simulink model "ASG_algorithm"  (R2024a)
settings: Solver=ode1  StartTime=0.0  StopTime=60  FixedStep=0.01  RelTol=1e-3
libraries: simulink x3
(part 2 of 3)

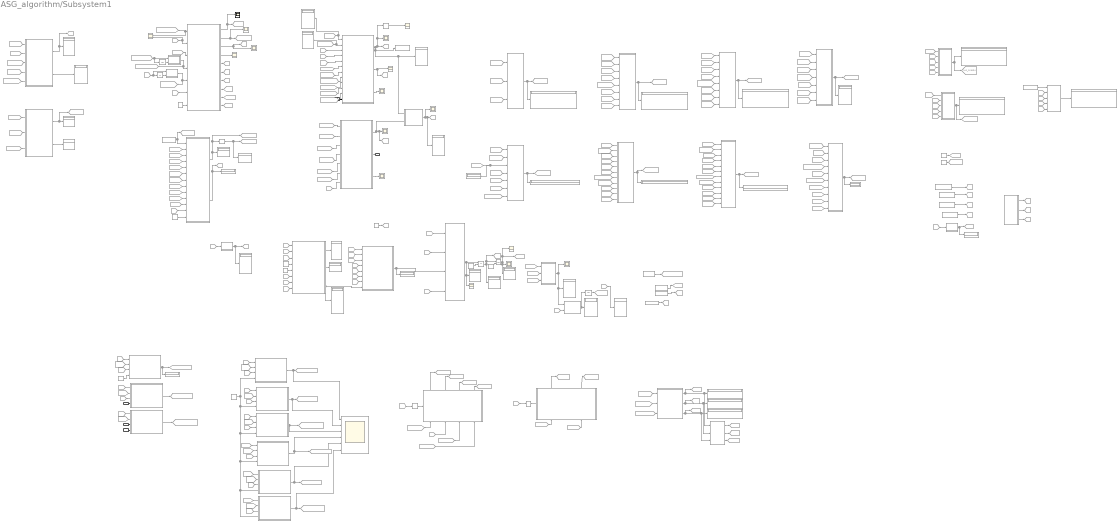
== system ASG_algorithm/Subsystem1 ==
  note: OMEGA DDOT
  note: K matrices
  note: INIT CONDITIONS
      | STEP31
  note: ETA 31
  note: DELTA 3.1
      | DELTA 3.1 DOT
  note: Av. SUBGRADIENT 31
  note: S1
  note: h0(omega_dot)
  note: S31
  note: h0(omega)
  note: CTES motor
  note: h0(x)
  note: ROTATION MATRIX R
  note: R 6x6
  note: THETA3 &
      | ALPHA
  note: DELTA 3.2
      | DELTA 3.2 DOT
  note: G312
  note: G322
  note: G311
  note: G310
  note: G313
  note: G321
  note: G320
  note: G323
  note: S32
  note: ETA 32
  note: INIT CONDITIONS
      | STEP31
  note: S3
  note: Av. SUBGRADIENT 32
  note: OMEGA DDOT
  note: gamma
  note: h3
  note: cte K3
  note: Q constructed
  note: OMEGA DOT
  note: OMEGA
  alpha : Inport
  constant sign : Inport  Port=2
  t : Inport  Port=3
  constant sign1 : Inport  Port=4
  A3 : Scope  Commented=on
  AVERAGE 3 BLOCK : Scope  Commented=on  NumInputPorts=6
  AverageBlock10 : Subsystem  Commented=on
  AverageBlock11 : Subsystem  Commented=on
  AverageBlock12 : Subsystem  Commented=on
  AverageBlock13 : Subsystem  Commented=on
  AverageBlock14 : Subsystem  Commented=on
  AverageBlock6 : Subsystem  Commented=on
  AverageBlock7 : Subsystem  Commented=on
  AverageBlock8 : Subsystem  Commented=on
  AverageBlock9 : Subsystem  Commented=on
  Compare To Constant1 : simulink/Logic and Bit Operations/Compare To Constant  Commented=on  relop===  const=0.0  OutDataTypeStr=boolean
  Compare To Constant2 : simulink/Logic and Bit Operations/Compare To Constant  Commented=on  relop===  const=0.0  OutDataTypeStr=boolean
  Constant11 : Constant  Commented=on  Value=0.5
  Constant12 : Constant  Commented=on  Value=[0;0;0;0;0;0]
  Constant13 : Constant  Commented=on  Value=353
  Constant14 : Constant  Commented=on  Value=2*10^(-4)
  Constant15 : Constant  Commented=on  Value=1.95*10^(-4)  VectorParams1D=off
  Constant17 : Constant  Commented=on  Value=0
  Constant18 : Constant  Commented=on  Value=10
  Constant19 : Constant  Commented=on  Value=[0;0;7;0;0;0]
  Constant{2,6,22,24} (4 alike) : Constant  Commented=on
  Constant20 : Constant  Commented=on  Value=0.00001
  Constant21 : Constant  Commented=on  Value=[0;0;0;0]
  Constant23 : Constant  Commented=on  Value=[1;1;1;1]
  Constant25 : Constant  Commented=on  Value=[0;0;1;0;0;0]
  Constant26 : Constant  Commented=on  Value=[1;1;1;1]
  Constant3 : Constant  Commented=on  Value=[0;0;0;0]
  Constant5 : Constant  Commented=on  Value=[0.1;0.1;0.1;0.1]
  Constant7 : Constant  Commented=on  Value=5*10^(-8)
  Constant8 : Constant  Commented=on  Value=0.01
  DELTA 31 : Scope
  DELTA31 DOT : Scope  Commented=on
  Derivative : Derivative  Commented=on
  Display{8,15,22,32,34,37,44..50,54..63,66,72,76,79..88,90..92} (39 alike) : Display  Commented=on
  Enabled Subsystem1 : Subsystem  Commented=on  TreatAsAtomicUnit=on
  Enabled Subsystem2 : Subsystem  Commented=on  TreatAsAtomicUnit=on
  From1 : From  Commented=on  GotoTag=QACT0
  From{124,128,194,227,236,249,277,326} (8 alike) : From  Commented=on  GotoTag=R6
  From{127,180,188,228,237,250,278,308} (8 alike) : From  Commented=on  GotoTag=H0_OMEGA
  From129 : From  Commented=on  GotoTag=QDES0
  From143 : From  Commented=on  GotoTag=QDOT_DES0
  From{144,151,154,160,166,173,176,185,191,198,220,242,253,265,287,293..294,301,303} (19 alike) : From  Commented=on  GotoTag=THETA3
  From145 : From  Commented=on  GotoTag=EPSILON
  From149 : From  Commented=on  GotoTag=A3_X
  From{150,153,159,167..168,172,175,183,190,201,240,243,254,266,286,292,296,304} (18 alike) : From  Commented=on  GotoTag=TIME
  From152 : From  Commented=on  GotoTag=A3_Y
  From155 : From  Commented=on  GotoTag=A3_Z
  From{156,169,200,280,310} (5 alike) : From  Commented=on  GotoTag=Q
  From158 : From  Commented=on  GotoTag=ETA3
  From161 : From  Commented=on  GotoTag=A3X_AVERAGE
  From162 : From  Commented=on  GotoTag=A3Y_AVERAGE
  From163 : From  Commented=on  GotoTag=A3Z_AVERAGE
  From164 : From  Commented=on  GotoTag=DELTA31
  From165 : From  Commented=on  GotoTag=DELTA31_DOT
  From170 : From  Commented=on  GotoTag=Q_DOT_STAR
  From171 : From  Commented=on  GotoTag=A3_PHI
  From174 : From  Commented=on  GotoTag=A3_THETA
  From177 : From  Commented=on  GotoTag=A3PHI_AVERAGE
  From178 : From  Commented=on  GotoTag=A3THETA_AVERAGE
  From179 : From  Commented=on  GotoTag=A3PSI_AVERAGE
  From18 : From  Commented=on  GotoTag=ANGLES_Q_DOT
  From{2,181,189,196,230,244,276,305} (8 alike) : From  Commented=on  GotoTag=KV
  From182 : From  Commented=on  GotoTag=H0_OMEGA_DOT
  From{184,192,241,252} (4 alike) : From  Commented=on  GotoTag=R6_DOT
  From186 : From  Commented=on  GotoTag=MIU
  From187 : From  Commented=on  GotoTag=R6_DDOT
  From193 : From  Commented=on  GotoTag=MIU
  From195 : From  Commented=on  GotoTag=MIU
  From197 : From  Commented=on  GotoTag=DELTA31
  From199 : From  Commented=on  GotoTag=JM
  From202 : From  Commented=on  GotoTag=K11
  From203 : From  Commented=on  GotoTag=K22
  From204 : From  Commented=on  GotoTag=K33
  From205 : From  Commented=on  GotoTag=L_ARM
  From206 : From  Commented=on  GotoTag=K11
  From207 : From  Commented=on  GotoTag=K22
  From208 : From  Commented=on  GotoTag=A3_PSI
  From209 : From  Commented=on  GotoTag=K33
  From210 : From  Commented=on  GotoTag=L_ARM
  From211 : From  Commented=on  GotoTag=U3_DOT
  From212 : From  Commented=on  GotoTag=K11
  From213 : From  Commented=on  GotoTag=K22
  From214 : From  Commented=on  GotoTag=K33
  From215 : From  Commented=on  GotoTag=L_ARM
  From216 : From  Commented=on  GotoTag=U3
  From221 : From  Commented=on  GotoTag=ZETA3
  From222 : From  Commented=on  GotoTag=ETA3
  From{223,233,245,258} (4 alike) : From  Commented=on  GotoTag=Z_VECTOR
  From{224,234,246,262,271} (5 alike) : From  Commented=on  GotoTag=D_INV
  From{225,235,248,263,272} (5 alike) : From  Commented=on  GotoTag=C_q
  From226 : From  Commented=on  GotoTag=THETA_ACTUAL
  From{229,238,251,264,273} (5 alike) : From  Commented=on  GotoTag=DRAG_MATRIX
  From239 : From  Commented=on  GotoTag=H0_OMEGA_DOT
  From247 : From  Commented=on  GotoTag=Q_ACTUAL
  From255 : From  Commented=on  GotoTag=Q_ACTUAL
  From256 : From  Commented=on  GotoTag=R6_DDOT
  From{257,267,289..290,313} (5 alike) : From  Commented=on  GotoTag=ALPHA
  From259 : From  Commented=on  GotoTag=Q_ACTUAL
  From260 : From  Commented=on  GotoTag=S3
  From261 : From  Commented=on  GotoTag=QDOT_ACTUAL
  From268 : From  Commented=on  GotoTag=q_dot_signal
  From269 : From  Commented=on  GotoTag=G_Q
  From270 : From  Commented=on  GotoTag=ETA3
  From274 : From  Commented=on  GotoTag=q_dot_signal
  From275 : From  Commented=on  GotoTag=G_Q
  From279 : From  Commented=on  GotoTag=U3
  From281 : From  Commented=on  GotoTag=EPSILON
  From283 : From  Commented=on  GotoTag=DELTA32
  From284 : From  Commented=on  GotoTag=DELTA32_DOT
  From285 : From  Commented=on  GotoTag=ETA32
  From288 : From  Commented=on  GotoTag=X32_AVG
  From291 : From  Commented=on  GotoTag=A32_X
  From295 : From  Commented=on  GotoTag=A32_Y
  From297 : From  Commented=on  GotoTag=DELTA32
  From298 : From  Commented=on  GotoTag=DELTA32_DOT
  From299 : From  Commented=on  GotoTag=DELTA32_DOT_0
  From300 : From  Commented=on  GotoTag=DELTA32_0
  From302 : From  Commented=on  GotoTag=A32_Z
  From306 : From  Commented=on  GotoTag=G322
  From307 : From  Commented=on  GotoTag=G312
  From309 : From  Commented=on  GotoTag=U3
  From314 : From  Commented=on  GotoTag=N3
  From315 : From  Commented=on  GotoTag=G310
  From316 : From  Commented=on  GotoTag=G313
  From317 : From  Commented=on  GotoTag=K3
  From318 : From  Commented=on  GotoTag=S31
  From319 : From  Commented=on  GotoTag=G321
  From320 : From  Commented=on  GotoTag=G320
  From321 : From  Commented=on  GotoTag=G323
  From322 : From  Commented=on  GotoTag=G312
  From323 : From  Commented=on  GotoTag=G322
  From324 : From  Commented=on  GotoTag=S32
  From325 : From  Commented=on  GotoTag=S3
  From327 : From  Commented=on  GotoTag=N3
  From36 : From  Commented=on  GotoTag=ANGLES_Q_DDOT
  From6 : From  Commented=on  GotoTag=G311
  From7 : From  Commented=on  GotoTag=QDOTACT0
  Goto100 : Goto  Commented=on  GotoTag=K11
  Goto101 : Goto  Commented=on  GotoTag=K22
  Goto102 : Goto  Commented=on  GotoTag=K33
  Goto103 : Goto  Commented=on  GotoTag=DM
  Goto104 : Goto  Commented=on  GotoTag=JM
  Goto105 : Goto  Commented=on  GotoTag=JM_INV
  Goto106 : Goto  Commented=on  GotoTag=DELTA32
  Goto107 : Goto  Commented=on  GotoTag=DELTA32_DOT
  Goto108 : Goto  Commented=on  GotoTag=QDOT_DES0
  Goto109 : Goto  Commented=on  GotoTag=ETA32
  Goto110 : Goto  Commented=on  GotoTag=DELTA32_0
  Goto111 : Goto  Commented=on  GotoTag=QDOTACT0
  Goto112 : Goto  Commented=on  GotoTag=QDES0
  Goto113 : Goto  Commented=on  GotoTag=DELTA32_DOT_0
  Goto114 : Goto  Commented=on  GotoTag=X32_AVG
  Goto115 : Goto  Commented=on  GotoTag=Y32_AVG
  Goto116 : Goto  Commented=on  GotoTag=Z32_AVG
  Goto117 : Goto  Commented=on  GotoTag=QDOT_ACTUAL
  Goto118 : Goto  Commented=on  GotoTag=QACT0
  Goto119 : Goto  Commented=on  GotoTag=A3PHI_AVERAGE
  Goto12 : Goto  Commented=on  GotoTag=Q
  Goto120 : Goto  Commented=on  GotoTag=A3THETA_AVERAGE
  Goto121 : Goto  Commented=on  GotoTag=A3PSI_AVERAGE
  Goto122 : Goto  Commented=on  GotoTag=A32_X
  Goto123 : Goto  Commented=on  GotoTag=U3_DOT
  Goto124 : Goto  Commented=on  GotoTag=U3
  Goto125 : Goto  Commented=on  GotoTag=Q_ACTUAL
  Goto126 : Goto  Commented=on  GotoTag=G312
  Goto127 : Goto  Commented=on  GotoTag=G311
  Goto128 : Goto  Commented=on  GotoTag=G310
  Goto129 : Goto  Commented=on  GotoTag=G313
  Goto13 : Goto  Commented=on  GotoTag=ETA3
  Goto130 : Goto  Commented=on  GotoTag=G322
  Goto131 : Goto  Commented=on  GotoTag=G321
  Goto132 : Goto  Commented=on  GotoTag=G320
  Goto133 : Goto  Commented=on  GotoTag=G323
  Goto134 : Goto  Commented=on  GotoTag=K3
  Goto135 : Goto  Commented=on  GotoTag=Q_ACTUAL
  Goto136 : Goto  Commented=on  GotoTag=S32
  Goto137 : Goto  Commented=on  GotoTag=S3
  Goto145 : Goto  Commented=on  GotoTag=Z_VECTOR
  Goto146 : Goto  Commented=on  GotoTag=N3
  Goto19 : Goto  Commented=on  GotoTag=ZETA3
  Goto20 : Goto  Commented=on  GotoTag=R6_DOT
  Goto27 : Goto  Commented=on  GotoTag=U3_DOT
  Goto33 : Goto  Commented=on  GotoTag=Q_DOT_STAR
  Goto34 : Goto  Commented=on  GotoTag=R6_DDOT
  Goto42 : Goto  Commented=on  GotoTag=A3_X
  Goto62 : Goto  Commented=on  GotoTag=R3
  Goto71 : Goto  Commented=on  GotoTag=A3_Y
  Goto77 : Goto  Commented=on  GotoTag=A3_Z
  Goto78 : Goto  Commented=on  GotoTag=A3
  Goto79 : Goto  Commented=on  GotoTag=DELTA31
  Goto8 : Goto  Commented=on  GotoTag=R6
  Goto80 : Goto  Commented=on  GotoTag=DELTA31_DOT
  Goto81 : Goto  Commented=on  GotoTag=H0_OMEGA
  Goto82 : Goto  Commented=on  GotoTag=S31
  Goto84 : Goto  Commented=on  GotoTag=H0_OMEGA_DOT
  Goto85 : Goto  Commented=on  GotoTag=THETA3
  Goto87 : Goto  Commented=on  GotoTag=R3_DOT
  Goto88 : Goto  Commented=on  GotoTag=R3_DDOT
  Goto89 : Goto  Commented=on  GotoTag=A3X_AVERAGE
  Goto90 : Goto  Commented=on  GotoTag=A3Y_AVERAGE
  Goto91 : Goto  Commented=on  GotoTag=A3Z_AVERAGE
  Goto92 : Goto  Commented=on  GotoTag=A3_PHI
  Goto93 : Goto  Commented=on  GotoTag=A3_THETA
  Goto94 : Goto  Commented=on  GotoTag=A3_PSI
  Goto96 : Goto  Commented=on  GotoTag=U3
  Goto97 : Goto  Commented=on  GotoTag=ALPHA
  Goto98 : Goto  Commented=on  GotoTag=KV
  Goto99 : Goto  Commented=on  GotoTag=KM
  Integrator7 : Integrator  Commented=on  InitialConditionSource=external  LimitOutput=on  UpperSaturationLimit=1000  LowerSaturationLimit=-1000
  Integrator8 : Integrator  Commented=on  InitialConditionSource=external  LimitOutput=on  UpperSaturationLimit=3200  LowerSaturationLimit=-3200
  MATLAB Function1 : MATLAB Function  Commented=on  TreatAsAtomicUnit=on
  MATLAB Function13 : MATLAB Function  Commented=on  TreatAsAtomicUnit=on
  MATLAB Function15 : MATLAB Function  Commented=on  TreatAsAtomicUnit=on
  MATLAB Function2 : MATLAB Function  Commented=on  TreatAsAtomicUnit=on
  MATLAB Function22 : MATLAB Function  Commented=on  TreatAsAtomicUnit=on
  MATLAB Function23 : MATLAB Function  Commented=on  TreatAsAtomicUnit=on
  MATLAB Function24 : MATLAB Function  Commented=on  TreatAsAtomicUnit=on
  MATLAB Function25 : MATLAB Function  Commented=on  TreatAsAtomicUnit=on
  MATLAB Function26 : MATLAB Function  Commented=on  TreatAsAtomicUnit=on
  MATLAB Function27 : MATLAB Function  Commented=on  TreatAsAtomicUnit=on
  MATLAB Function29 : MATLAB Function  Commented=on  TreatAsAtomicUnit=on
  MATLAB Function30 : MATLAB Function  Commented=on  TreatAsAtomicUnit=on
  MATLAB Function31 : MATLAB Function  Commented=on  TreatAsAtomicUnit=on
  MATLAB Function32 : MATLAB Function  Commented=on  TreatAsAtomicUnit=on
  MATLAB Function33 : MATLAB Function  Commented=on  TreatAsAtomicUnit=on
  MATLAB Function34 : MATLAB Function  Commented=on  TreatAsAtomicUnit=on
  MATLAB Function35 : MATLAB Function  Commented=on  TreatAsAtomicUnit=on
  MATLAB Function36 : MATLAB Function  Commented=on  TreatAsAtomicUnit=on
  MATLAB Function37 : MATLAB Function  Commented=on  TreatAsAtomicUnit=on
  MATLAB Function38 : MATLAB Function  Commented=on  TreatAsAtomicUnit=on
  MATLAB Function39 : MATLAB Function  Commented=on  TreatAsAtomicUnit=on
  MATLAB Function40 : MATLAB Function  Commented=on  TreatAsAtomicUnit=on
  MATLAB Function41 : MATLAB Function  Commented=on  TreatAsAtomicUnit=on
  MATLAB Function42 : MATLAB Function  Commented=on  TreatAsAtomicUnit=on
  MATLAB Function43 : MATLAB Function  Commented=on  TreatAsAtomicUnit=on
  MATLAB Function44 : MATLAB Function  Commented=on  TreatAsAtomicUnit=on
  MATLAB Function46 : MATLAB Function  Commented=on  TreatAsAtomicUnit=on
  MATLAB Function47 : MATLAB Function  Commented=on  TreatAsAtomicUnit=on
  NORM S3 : Scope  Commented=on
  NORM S32 : Scope  Commented=on
  Norm D3 : Scope  Commented=on
  OMEGA DDOT : Scope  Commented=on
  Q constructed : Scope  Commented=on
  S3 GRAL : Scope  Commented=on
  S31 6X1 : Scope  Commented=on
  "S32 3X1 " : Scope  Commented=on
  SIGN S3 : Scope  Commented=on
  Scope : Scope  Commented=on
  Scope5 : Scope  Commented=on
  Sign : Signum  Commented=on
  To Workspace12 : ToWorkspace  Commented=on  VariableName=s3  SampleTime=-1
  Unit Delay : UnitDelay  Commented=on  SampleTime=-1  HasFrameUpgradeWarning=on
  Unit Delay1 : UnitDelay  Commented=on  SampleTime=0.01  HasFrameUpgradeWarning=on
  Unit Delay2 : UnitDelay  Commented=on  SampleTime=0.01  HasFrameUpgradeWarning=on
  ZETA3 : Scope  Commented=on
  compare Q : Scope  Commented=on  NumInputPorts=2
  eta3 : MATLAB Function  Commented=on  TreatAsAtomicUnit=on
  eta4 : MATLAB Function  Commented=on  TreatAsAtomicUnit=on
  Z32 : Outport
  wires:
  Constant12/1 -> Goto125/1
  MATLAB Function2/3(R_ddot) -> Goto88/1, MATLAB Function13/3(R_ddot), Display50/1
  Enabled Subsystem2/1(delta32_0) -> Goto110/1
  From272/1 -> MATLAB Function22/3(C)
  From222/1 -> MATLAB Function32/7(eta3)
  From262/1 -> MATLAB Function36/2(D_inv)
  Constant20/1 -> Goto99/1
  MATLAB Function22/2(a3) -> Goto122/1, Display76/1
  MATLAB Function23/1(G322) -> Goto126/1, Display22/1
  From176/1 -> AverageBlock11/2(theta)
  From243/1 -> MATLAB Function34/11(t)
  Integrator7/1 -> Goto27/1, Integrator8/1, Display85/1
  From304/1 -> AverageBlock12/3(t)
  MATLAB Function13/1(R_six) -> Goto8/1
  Compare To Constant1/1 -> Enabled Subsystem1/Enable
  Enabled Subsystem1/1(Q_actual0) -> Goto118/1
  From254/1 -> MATLAB Function35/10(t)
  From158/1 -> MATLAB Function15/3(eta3)
  From324/1 -> MATLAB Function42/6(s32)
  Compare To Constant2/1 -> Enabled Subsystem2/Enable
  Constant8/1 -> Goto85/1
  Constant5/1 -> MATLAB Function24/1(x)
  From253/1 -> MATLAB Function35/9(theta3)
  From124/1 -> MATLAB Function23/2(R6)
  From197/1 -> MATLAB Function32/1(delta31)
  From144/1 -> eta3/1(theta3)
  From275/1 -> MATLAB Function22/6(G_q)
  From230/1 -> MATLAB Function34/1(Kv)
  From280/1 -> MATLAB Function40/1(u), Unit Delay2/1
  Derivative/1 -> Display62/1, Goto107/1
  MATLAB Function43/3(h3) -> MATLAB Function42/8(h3), Display82/1
  MATLAB Function34/1(G321) -> Goto131/1, Display54/1
  From167/1 -> AverageBlock6/3(t)
  From265/1 -> MATLAB Function36/5(theta3)
  From313/1 -> MATLAB Function37/7(alpha)
  Constant22/1 -> AverageBlock6/4(constant sign), AverageBlock8/4(constant sign), AverageBlock11/4(constant sign), AverageBlock10/4(constant sign), AverageBlock9/4(constant sign), AverageBlock7/4(constant sign)
  From327/1 -> MATLAB Function42/1(n3)
  Enabled Subsystem1/2(Q_desired0) -> Goto112/1
  From246/1 -> MATLAB Function35/3(D_inv)
  Constant17/1 -> Integrator7/2
  From248/1 -> MATLAB Function35/4(C)
  From244/1 -> MATLAB Function35/1(Kv)
  From268/1 -> MATLAB Function36/8(q_dot)
  From128/1 -> MATLAB Function30/2(R6)
  Unit Delay1/1 -> MATLAB Function39/2(u_delay)
  From143/1 -> eta3/5(Qdotdesired_0)
  Enabled Subsystem1/3(Qdot_actual0) -> Goto111/1
  MATLAB Function15/3(norm_s3) -> NORM S3/1
  Constant11/1 -> Goto97/1
  From319/1 -> MATLAB Function43/6(G321)
  From192/1 -> MATLAB Function31/4(R6_dot)
  From263/1 -> MATLAB Function36/3(C)
  From256/1 -> MATLAB Function35/11(R6_ddot)
  From161/1 -> MATLAB Function15/6(a3x_average)
  Constant7/1 -> Goto98/1
  From156/1 -> compare Q/2, MATLAB Function1/2(Q_desired)
  From259/1 -> Enabled Subsystem1/1(Q_actual)
  From298/1 -> Enabled Subsystem2/2(delta32_dot)
  MATLAB Function43/2(h32) -> Display81/1
  From250/1 -> MATLAB Function35/6(h0_omega)
  From286/1 -> MATLAB Function37/4(t)
  Constant3/1 -> Goto123/1
  From285/1 -> MATLAB Function37/3(eta32)
  From257/1 -> MATLAB Function35/12(alpha)
  AverageBlock10/1(Out1) -> AVERAGE 3 BLOCK/5, Goto120/1
  From223/1 -> MATLAB Function34/2(z_vector)
  From269/1 -> MATLAB Function36/9(G_q)
  From291/1 -> AverageBlock12/1(a3_x)
  From206/1 -> MATLAB Function25/2(K11)
  From162/1 -> MATLAB Function15/7(a3y_average)
  From36/1 -> MATLAB Function2/3(anglesddot_vector)
  MATLAB Function22/1(delta32) -> Derivative/1, Goto106/1, Display61/1
  From255/1 -> Unit Delay1/1, MATLAB Function39/1(u)
  From240/1 -> AverageBlock9/3(t)
  MATLAB Function40/1(derivada) -> Goto33/1, MATLAB Function1/5(Qdot_desired)
  AverageBlock9/1(Out1) -> AVERAGE 3 BLOCK/4, Goto119/1
  From168/1 -> Compare To Constant1/1
  From281/1 -> MATLAB Function22/11(epsilon)
  From260/1 -> MATLAB Function47/1(s3)
  From220/1 -> AverageBlock9/2(theta)
  From276/1 -> MATLAB Function22/7(Kv)
  From154/1 -> AverageBlock8/2(theta)
  MATLAB Function27/1(h_x) -> Goto84/1, Display58/1
  MATLAB Function1/1(delta3) -> DELTA 31/1, Goto79/1
  AverageBlock8/1(Out1) -> AVERAGE 3 BLOCK/3, Goto91/1
  From234/1 -> MATLAB Function34/3(D_inv)
  From239/1 -> MATLAB Function34/8(h0_omegadot)
  From322/1 -> MATLAB Function42/4(G312)
  From155/1 -> AverageBlock8/1(In1)
  MATLAB Function15/1(s3) -> Sign/1, S31 6X1/1, Goto82/1, MATLAB Function38/1(S31), Display32/1, To Workspace12/1
  From181/1 -> MATLAB Function30/1(Kv)
  MATLAB Function42/1(gamma) -> Display83/1, MATLAB Function41/3(gamma)
  AverageBlock11/1(Out1) -> AVERAGE 3 BLOCK/6, Goto121/1
  From160/1 -> MATLAB Function15/5(theta3)
  MATLAB Function15/2(Z3) -> ZETA3/1, Goto19/1
  From316/1 -> MATLAB Function43/3(G313)
  MATLAB Function36/1(G323) -> Goto133/1, Display60/1
  AverageBlock7/1(Out1) -> Goto90/1, AVERAGE 3 BLOCK/2
  MATLAB Function44/1(y) -> MATLAB Function46/1(Fb), Display87/1, Q constructed/1
  eta3/2(sum_result) -> Display15/1
  MATLAB Function24/1(h_x) -> Display56/1
  From261/1 -> Enabled Subsystem1/3(Qdot_actual)
  From205/1 -> MATLAB Function24/5(larm)
  MATLAB Function1/5(a3_x) -> Goto42/1
  MATLAB Function1/9(a3_theta) -> Goto93/1
  Constant26/1 -> Goto124/1
  From210/1 -> MATLAB Function25/5(larm)
  From297/1 -> Enabled Subsystem2/1(delta32)
  From149/1 -> AverageBlock6/1(a3_x)
  From172/1 -> AverageBlock10/3(t)
  From203/1 -> MATLAB Function24/3(K22)
  From209/1 -> MATLAB Function25/4(K33)
  eta4/1(eta3) -> Goto109/1, Display66/1
  MATLAB Function33/2(K22) -> Goto101/1
  MATLAB Function25/1(h_x) -> Goto81/1, Display57/1
  From129/1 -> eta3/3(Qdesired_0)
  MATLAB Function37/3(norm_s3) -> NORM S32/1
  From224/1 -> Display92/1, MATLAB Function29/3(D_inv)
  MATLAB Function1/4(F_d3) -> Norm D3/1
  From177/1 -> MATLAB Function15/9(a3phi_average)
  From325/1 -> MATLAB Function42/2(s3)
  From303/1 -> AverageBlock12/2(theta)
  Enabled Subsystem1/4(Qdot_desired0) -> Goto108/1
  MATLAB Function29/1(G322) -> Goto130/1, Display48/1
  From165/1 -> Display34/1, MATLAB Function15/2(delta3_dot)
  From152/1 -> AverageBlock7/1(In1)
  From178/1 -> MATLAB Function15/10(a3theta_average)
  From274/1 -> MATLAB Function22/5(q_dot_signal)
  From184/1 -> MATLAB Function30/4(R6_dot)
  MATLAB Function2/1(R) -> Goto62/1, MATLAB Function13/1(R), Display44/1
  From164/1 -> MATLAB Function15/1(delta3), Display37/1
  Constant15/1 -> Goto104/1
  From214/1 -> MATLAB Function27/4(K33)
  From166/1 -> AverageBlock6/2(theta)
  From201/1 -> MATLAB Function32/3(t)
  From213/1 -> MATLAB Function27/3(K22)
  From242/1 -> MATLAB Function34/10(theta3)
  From198/1 -> MATLAB Function32/4(theta3)
  MATLAB Function37/2(Z32) -> Z32/1
  From153/1 -> AverageBlock8/3(t)
  From171/1 -> AverageBlock9/1(a3_x)
  MATLAB Function1/3(a3) -> Goto78/1, A3/1
  From305/1 -> MATLAB Function44/3(kv)
  From145/1 -> MATLAB Function1/3(epsilon)
  MATLAB Function33/3(K33) -> Goto102/1
  From207/1 -> MATLAB Function25/3(K22)
  Integrator8/1 -> Scope/1, Goto96/1, Display86/1, Scope5/1
  From1/1 -> eta3/2(Qactual_0)
  From179/1 -> MATLAB Function15/11(a3psi_average)
  From175/1 -> AverageBlock11/3(t)
  From200/1 -> MATLAB Function32/5(Q_deseada)
  MATLAB Function38/1(S3) -> S3 GRAL/1, Goto137/1, Display72/1
  Constant2/1 -> MATLAB Function22/13(k32)
  From174/1 -> AverageBlock10/1(In1)
  MATLAB Function1/6(a3_y) -> Goto71/1
  MATLAB Function13/2(R_dotsix) -> Goto20/1
  Constant13/1 -> Integrator8/2
  From202/1 -> MATLAB Function24/2(K11)
  From296/1 -> Compare To Constant2/1
  From170/1 -> Enabled Subsystem1/4(Qdot_desired)
  MATLAB Function1/2(delta3_dot) -> DELTA31 DOT/1, Goto80/1
  From267/1 -> MATLAB Function36/7(alpha)
  From279/1 -> MATLAB Function22/10(omega_vector)
  MATLAB Function30/1(G311) -> Goto127/1, Display45/1
  From284/1 -> MATLAB Function37/2(delta32_dot)
  From159/1 -> MATLAB Function15/4(t)
  MATLAB Function1/7(a3_z) -> Goto77/1
  From277/1 -> MATLAB Function22/8(R6)
  From191/1 -> MATLAB Function31/6(theta3)
  From18/1 -> MATLAB Function2/2(anglesdot_vector)
  From196/1 -> MATLAB Function29/1(Kv)
  MATLAB Function37/1(s32) -> MATLAB Function38/2(S32), "S32 3X1 "/1, Goto136/1
  MATLAB Function39/1(derivada) -> Goto117/1, MATLAB Function1/4(Qdot_actual)
  Constant23/1 -> MATLAB Function43/5(omega)
  alpha/1 -> MATLAB Function15/12(alpha)
  From211/1 -> MATLAB Function27/1(x)
  Constant18/1 -> MATLAB Function1/7(k31)
  From245/1 -> MATLAB Function36/1(z_vector)
  MATLAB Function1/8(a3_phi) -> Goto92/1
  From127/1 -> MATLAB Function23/3(h0_omega)
  From252/1 -> MATLAB Function35/8(R6_dot)
  From193/1 -> MATLAB Function31/7(miu)
  From185/1 -> MATLAB Function30/7(theta3)
  From189/1 -> MATLAB Function31/1(Kv)
  AverageBlock14/1(Out1) -> Goto116/1
  From183/1 -> MATLAB Function30/6(t)
  From293/1 -> AverageBlock13/2(theta)
  From182/1 -> MATLAB Function30/5(h0_omegadot)
  Constant24/1 -> Goto134/1
  From241/1 -> MATLAB Function34/9(R6_dot)
  From195/1 -> MATLAB Function32/2(miu)
  Constant25/1 -> Goto145/1, MATLAB Function22/1(z_vector)
  From194/1 -> MATLAB Function31/8(R6)
  From199/1 -> MATLAB Function26/1(Jm)
  From237/1 -> MATLAB Function34/6(h0_omega)
  From212/1 -> MATLAB Function27/2(K11)
  From270/1 -> MATLAB Function36/10(eta3)
  From221/1 -> MATLAB Function32/6(zeta3)
  MATLAB Function32/1(G313) -> Goto129/1, Display47/1
  From163/1 -> MATLAB Function15/8(a3z_average)
  MATLAB Function33/1(K11) -> Goto100/1
  From208/1 -> AverageBlock11/1(In1)
  From292/1 -> AverageBlock13/3(t)
  MATLAB Function1/10(a3_psi) -> Goto94/1
  Constant14/1 -> Goto103/1
  constant sign/1 -> AverageBlock13/4(constant sign)
  From228/1 -> MATLAB Function29/6(h0_omega)
  From320/1 -> MATLAB Function43/7(G320)
  From287/1 -> MATLAB Function37/5(theta3)
  From301/1 -> AverageBlock14/2(theta)
  From247/1 -> compare Q/1, MATLAB Function1/1(Q_actual)
  MATLAB Function41/1(omegaddot) -> OMEGA DDOT/1, Display84/1, Integrator7/1
  From302/1 -> AverageBlock14/1(In1)
  From295/1 -> AverageBlock13/1(In1)
  From225/1 -> MATLAB Function29/4(C)
  From235/1 -> MATLAB Function34/4(C)
  Unit Delay2/1 -> MATLAB Function40/2(u_delay)
  MATLAB Function26/1(Jm_inv) -> Goto105/1, Display55/1
  From226/1 -> MATLAB Function2/1(angles_vector)
  From236/1 -> MATLAB Function34/5(R6)
  eta3/1(eta3) -> Goto13/1, Display8/1
  From238/1 -> MATLAB Function34/7(drag_matrix)
  Constant6/1 -> AverageBlock12/4(constant sign)
  From6/1 -> MATLAB Function43/1(G311)
  From307/1 -> MATLAB Function41/1(G312)
  From308/1 -> MATLAB Function44/1(h0_omega)
  From151/1 -> AverageBlock7/2(theta)
  From309/1 -> MATLAB Function44/2(omega)
  Sign/1 -> SIGN S3/1
  From180/1 -> MATLAB Function30/3(h0_omega)
  From278/1 -> MATLAB Function22/9(h0_omega)
  From173/1 -> AverageBlock10/2(theta)
  From188/1 -> MATLAB Function31/3(h0_omega)
  From288/1 -> MATLAB Function37/6(a3x_average)
  From258/1 -> MATLAB Function29/2(z_vector)
  From251/1 -> MATLAB Function35/7(drag_matrix)
  From187/1 -> MATLAB Function31/2(R6_ddot)
  From283/1 -> MATLAB Function37/1(delta32)
  From229/1 -> MATLAB Function29/7(drag_matrix)
  eta4/2(sum_result) -> Display63/1
  From323/1 -> MATLAB Function42/7(G322)
  From299/1 -> eta4/3(delta32_dot0)
  From300/1 -> eta4/2(delta32_0)
  From204/1 -> MATLAB Function24/4(K33)
  AverageBlock6/1(Out1) -> Goto89/1, AVERAGE 3 BLOCK/1
  Enabled Subsystem2/2(delta32_dot_0) -> Goto113/1
  From7/1 -> eta3/4(Qdotactual_0)
  MATLAB Function47/1(n3) -> Display91/1, Goto146/1
  AverageBlock13/1(Out1) -> Goto115/1
  From273/1 -> MATLAB Function22/4(drag_matrix)
  From215/1 -> MATLAB Function27/5(larm)
  From294/1 -> eta4/1(theta3)
  From169/1 -> Enabled Subsystem1/2(Q_desired)
  Constant21/1 -> MATLAB Function43/4(omega_dot)
  AverageBlock12/1(Out1) -> Display79/1, Goto114/1
  From318/1 -> MATLAB Function42/5(s31)
  From264/1 -> MATLAB Function36/4(drag_matrix)
  From315/1 -> MATLAB Function43/2(G310)
  MATLAB Function13/3(R_ddotsix) -> Goto34/1
  From186/1 -> MATLAB Function30/8(miu)
  t/1 -> AverageBlock14/3(t)
  From306/1 -> MATLAB Function41/2(G322)
  From216/1 -> MATLAB Function25/1(x)
  From314/1 -> MATLAB Function41/4(n3)
  MATLAB Function35/1(G320) -> Goto132/1, Display59/1
  MATLAB Function43/1(h31) -> Display80/1
  From150/1 -> AverageBlock7/3(t)
  From317/1 -> MATLAB Function42/3(k3)
  From190/1 -> MATLAB Function31/5(t)
  MATLAB Function2/2(R_dot) -> Goto87/1, MATLAB Function13/2(R_dot), Display49/1
  From233/1 -> MATLAB Function35/2(z_vector)
  From266/1 -> MATLAB Function36/6(t)
  From321/1 -> MATLAB Function43/8(G323)
  Constant19/1 -> Goto12/1
  From2/1 -> MATLAB Function23/1(Kv)
  From227/1 -> MATLAB Function29/5(R6)
  From271/1 -> MATLAB Function22/2(D_inv)
  From326/1 -> MATLAB Function46/2(R6)
  From310/1 -> Display88/1
  constant sign1/1 -> AverageBlock14/4(constant sign)
  From289/1 -> MATLAB Function22/12(alpha)
  MATLAB Function46/1(Q_costructed) -> Unit Delay/1, Display90/1
  Unit Delay/1 -> Goto135/1
  MATLAB Function31/1(G311) -> Goto128/1, Display46/1
  From290/1 -> MATLAB Function1/6(alpha)
  From249/1 -> MATLAB Function35/5(R6)

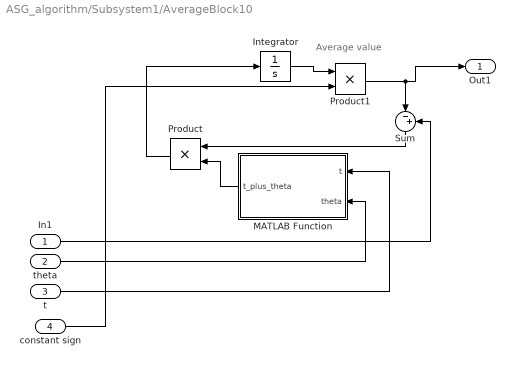
== system ASG_algorithm/Subsystem1/AverageBlock10 ==
  note: Average value
  In1 : Inport
  theta : Inport  Port=2
  t : Inport  Port=3
  constant sign : Inport  Port=4
  Integrator : Integrator
  MATLAB Function : MATLAB Function  TreatAsAtomicUnit=on
  Product : Product
  Product1 : Product
  Sum : Sum  Inputs=|-+
  Out1 : Outport
  wires:
  MATLAB Function/1(t_plus_theta) -> Product/2
  Sum/1 -> Product/1
  Product/1 -> Integrator/1
  theta/1 -> MATLAB Function/2(theta)
  In1/1 -> Sum/2
  t/1 -> MATLAB Function/1(t)
  Integrator/1 -> Product1/1
  Product1/1 -> Sum/1, Out1/1
  constant sign/1 -> Product1/2

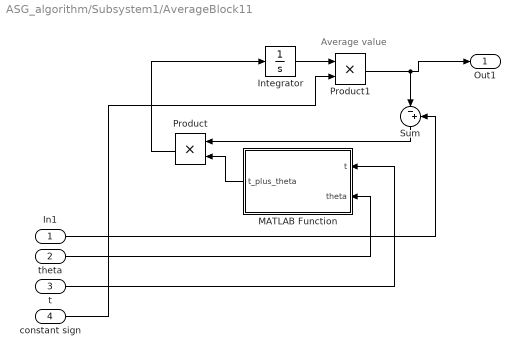
== system ASG_algorithm/Subsystem1/AverageBlock11 ==
  note: Average value
  In1 : Inport
  theta : Inport  Port=2
  t : Inport  Port=3
  constant sign : Inport  Port=4
  Integrator : Integrator
  MATLAB Function : MATLAB Function  TreatAsAtomicUnit=on
  Product : Product
  Product1 : Product
  Sum : Sum  Inputs=|-+
  Out1 : Outport
  wires:
  MATLAB Function/1(t_plus_theta) -> Product/2
  Sum/1 -> Product/1
  Product/1 -> Integrator/1
  theta/1 -> MATLAB Function/2(theta)
  In1/1 -> Sum/2
  t/1 -> MATLAB Function/1(t)
  Integrator/1 -> Product1/1
  Product1/1 -> Sum/1, Out1/1
  constant sign/1 -> Product1/2

== system ASG_algorithm/Subsystem1/AverageBlock12 ==
  note: Average value
  a3_x : Inport
  theta : Inport  Port=2
  t : Inport  Port=3
  constant sign : Inport  Port=4
  Integrator : Integrator
  MATLAB Function : MATLAB Function  TreatAsAtomicUnit=on
  Product : Product
  Product1 : Product
  Sum : Sum  Inputs=|-+
  Out1 : Outport
  wires:
  MATLAB Function/1(t_plus_theta) -> Product/2
  Sum/1 -> Product/1
  Product/1 -> Integrator/1
  theta/1 -> MATLAB Function/2(theta)
  a3_x/1 -> Sum/2
  t/1 -> MATLAB Function/1(t)
  Integrator/1 -> Product1/1
  constant sign/1 -> Product1/2
  Product1/1 -> Sum/1, Out1/1

== system ASG_algorithm/Subsystem1/AverageBlock13 ==
  note: Average value
  In1 : Inport
  theta : Inport  Port=2
  t : Inport  Port=3
  constant sign : Inport  Port=4
  Integrator : Integrator
  MATLAB Function : MATLAB Function  TreatAsAtomicUnit=on
  Product : Product
  Product1 : Product
  Sum : Sum  Inputs=|-+
  Out1 : Outport
  wires:
  MATLAB Function/1(t_plus_theta) -> Product/2
  Sum/1 -> Product/1
  Product/1 -> Integrator/1
  theta/1 -> MATLAB Function/2(theta)
  In1/1 -> Sum/2
  t/1 -> MATLAB Function/1(t)
  Integrator/1 -> Product1/1
  Product1/1 -> Sum/1, Out1/1
  constant sign/1 -> Product1/2

== system ASG_algorithm/Subsystem1/AverageBlock14 ==
  note: Average value
  In1 : Inport
  theta : Inport  Port=2
  t : Inport  Port=3
  constant sign : Inport  Port=4
  Integrator : Integrator
  MATLAB Function : MATLAB Function  TreatAsAtomicUnit=on
  Product : Product
  Product1 : Product
  Sum : Sum  Inputs=|-+
  Out1 : Outport
  wires:
  MATLAB Function/1(t_plus_theta) -> Product/2
  Sum/1 -> Product/1
  Product/1 -> Integrator/1
  theta/1 -> MATLAB Function/2(theta)
  In1/1 -> Sum/2
  t/1 -> MATLAB Function/1(t)
  Integrator/1 -> Product1/1
  Product1/1 -> Sum/1, Out1/1
  constant sign/1 -> Product1/2

== system ASG_algorithm/Subsystem1/AverageBlock6 ==
  note: Average value
  a3_x : Inport
  theta : Inport  Port=2
  t : Inport  Port=3
  constant sign : Inport  Port=4
  Integrator : Integrator
  MATLAB Function : MATLAB Function  TreatAsAtomicUnit=on
  Product : Product
  Product1 : Product
  Sum : Sum  Inputs=|-+
  Out1 : Outport
  wires:
  MATLAB Function/1(t_plus_theta) -> Product/2
  Sum/1 -> Product/1
  Product/1 -> Integrator/1
  theta/1 -> MATLAB Function/2(theta)
  a3_x/1 -> Sum/2
  t/1 -> MATLAB Function/1(t)
  Integrator/1 -> Product1/1
  constant sign/1 -> Product1/2
  Product1/1 -> Sum/1, Out1/1

== system ASG_algorithm/Subsystem1/AverageBlock7 ==
  note: Average value
  In1 : Inport
  theta : Inport  Port=2
  t : Inport  Port=3
  constant sign : Inport  Port=4
  Integrator : Integrator
  MATLAB Function : MATLAB Function  TreatAsAtomicUnit=on
  Product : Product
  Product1 : Product
  Sum : Sum  Inputs=|-+
  Out1 : Outport
  wires:
  MATLAB Function/1(t_plus_theta) -> Product/2
  Sum/1 -> Product/1
  Product/1 -> Integrator/1
  theta/1 -> MATLAB Function/2(theta)
  In1/1 -> Sum/2
  t/1 -> MATLAB Function/1(t)
  Integrator/1 -> Product1/1
  Product1/1 -> Sum/1, Out1/1
  constant sign/1 -> Product1/2

== system ASG_algorithm/Subsystem1/AverageBlock8 ==
  note: Average value
  In1 : Inport
  theta : Inport  Port=2
  t : Inport  Port=3
  constant sign : Inport  Port=4
  Integrator : Integrator
  MATLAB Function : MATLAB Function  TreatAsAtomicUnit=on
  Product : Product
  Product1 : Product
  Sum : Sum  Inputs=|-+
  Out1 : Outport
  wires:
  MATLAB Function/1(t_plus_theta) -> Product/2
  Sum/1 -> Product/1
  Product/1 -> Integrator/1
  theta/1 -> MATLAB Function/2(theta)
  In1/1 -> Sum/2
  t/1 -> MATLAB Function/1(t)
  Integrator/1 -> Product1/1
  Product1/1 -> Sum/1, Out1/1
  constant sign/1 -> Product1/2

== system ASG_algorithm/Subsystem1/AverageBlock9 ==
  note: Average value
  a3_x : Inport
  theta : Inport  Port=2
  t : Inport  Port=3
  constant sign : Inport  Port=4
  Integrator : Integrator
  MATLAB Function : MATLAB Function  TreatAsAtomicUnit=on
  Product : Product
  Product1 : Product
  Sum : Sum  Inputs=|-+
  Out1 : Outport
  wires:
  MATLAB Function/1(t_plus_theta) -> Product/2
  Sum/1 -> Product/1
  Product/1 -> Integrator/1
  theta/1 -> MATLAB Function/2(theta)
  a3_x/1 -> Sum/2
  t/1 -> MATLAB Function/1(t)
  Integrator/1 -> Product1/1
  constant sign/1 -> Product1/2
  Product1/1 -> Sum/1, Out1/1

== system ASG_algorithm/Subsystem1/Enabled Subsystem1 ==
  Q_actual : Inport
  Q_desired : Inport  Port=2
  Qdot_actual : Inport  Port=3
  Qdot_desired : Inport  Port=4
  Enable : EnablePort
  MATLAB Function : MATLAB Function  TreatAsAtomicUnit=on
  Q_actual0 : Outport
  Q_desired0 : Outport  Port=2
  Qdot_actual0 : Outport  Port=3
  Qdot_desired0 : Outport  Port=4
  wires:
  Q_actual/1 -> MATLAB Function/1(Q_actual)
  MATLAB Function/2(Qdesired_0) -> Q_desired0/1
  MATLAB Function/1(Qactual_0) -> Q_actual0/1
  MATLAB Function/3(Qdotactual_0) -> Qdot_actual0/1
  MATLAB Function/4(Qdotdesired_0) -> Qdot_desired0/1
  Q_desired/1 -> MATLAB Function/2(Q_desired)
  Qdot_actual/1 -> MATLAB Function/3(Qdot_actual)
  Qdot_desired/1 -> MATLAB Function/4(Qdot_desired)

== system ASG_algorithm/Subsystem1/Enabled Subsystem2 ==
  delta32 : Inport
  delta32_dot : Inport  Port=2
  Enable : EnablePort
  MATLAB Function : MATLAB Function  TreatAsAtomicUnit=on
  delta32_0 : Outport
  delta32_dot_0 : Outport  Port=2
  wires:
  delta32/1 -> MATLAB Function/1(delta32)
  MATLAB Function/2(delta32_dot_0) -> delta32_dot_0/1
  MATLAB Function/1(delta32_0) -> delta32_0/1
  delta32_dot/1 -> MATLAB Function/2(delta32_dot)

== matlab function ASG_algorithm/MATLAB Function3 ==
  data: kappa_actual input; delta1 output; delta1_dot output; a1 output; kappa_desired input; F_d1 output; epsilon input; v_actual input; v_desired input; a1_x output; a1_y output; a1_z output
function [delta1, delta1_dot,a1, F_d1, a1_x, a1_y, a1_z] = fcn(kappa_actual, kappa_desired,  epsilon, v_actual, v_desired)
delta1=kappa_actual-kappa_desired;
delta1_dot=v_actual-v_desired;
F_d1=norm(delta1);
if F_d1 < epsilon
    a1 = zeros(3,1);
else
a1 = -delta1;  %quite el signo /F_d1
end
a1_x = a1(1);
a1_y = a1(2);
a1_z = a1(3);

== matlab function ASG_algorithm/MATLAB Function4 ==
  data: xi_subkappa input; k1 output; xi_subkappa_dot input; t input; theta1 input; rho1 input
function k1 = fcn(xi_subkappa,xi_subkappa_dot, t,theta1,rho1 )
k1= norm(xi_subkappa)/(t+theta1)+norm(xi_subkappa_dot)+rho1;

== matlab function ASG_algorithm/MATLAB Function7 ==
  data: vector_rpy input; R_graph output
function R_graph= fcn(vector_rpy)
%Euler values to rotation matrix x,y,z 
R_graph=eul2rotm([vector_rpy(1) vector_rpy(2) vector_rpy(3)]);

== matlab function ASG_algorithm/AverageBlock3/MATLAB Function ==
  data: t input; t_plus_theta output; theta input
function t_plus_theta = fcn(t, theta)
t_plus_theta = 1/(t+theta);

== matlab function ASG_algorithm/AverageBlock4/MATLAB Function ==
  data: t input; t_plus_theta output; theta input
function t_plus_theta = fcn(t, theta)
t_plus_theta = 1/(t+theta);

== matlab function ASG_algorithm/AverageBlock/MATLAB Function ==
  data: t input; t_plus_theta output; theta input
function t_plus_theta = fcn(t, theta)
t_plus_theta = 1/(t+theta);

== matlab function ASG_algorithm/AverageBlock1/MATLAB Function ==
  data: t input; t_plus_theta output; theta input
function t_plus_theta = fcn(t, theta)
t_plus_theta = 1/(t+theta);

== matlab function ASG_algorithm/AverageBlock2/MATLAB Function ==
  data: t input; t_plus_theta output; theta input
function t_plus_theta = fcn(t, theta)
t_plus_theta = 1/(t+theta);

== matlab function ASG_algorithm/AverageBlock5/MATLAB Function ==
  data: t input; t_plus_theta output; theta input
function t_plus_theta = fcn(t, theta)
t_plus_theta = 1/(t+theta);

== matlab function ASG_algorithm/MATLAB Function16 ==
  data: fv input; hv output; v_dot_deseada input; v_actual input; v_deseada input; theta1 input; a1 input; eta1 input; delta1 input; zeta1 input; t input
function hv = fcn(fv,v_dot_deseada,v_actual, v_deseada,theta1,a1,eta1,delta1,zeta1,t)
hv= fv-v_dot_deseada+(v_actual-v_deseada)/(t+theta1) - a1/(t+theta1) - (delta1+eta1)/(t+theta1)^2 + zeta1/(t+theta1)^2;

== matlab function ASG_algorithm/eta1 ==
  data: theta1 input; eta1 output; v_0 input; v_deseada_0 input; kappa_desired_0 input; kappa_0 input; sum_result output
function [eta1, sum_result] = fcn(theta1,v_0, v_deseada_0, kappa_desired_0, kappa_0)
eta1 = -theta1*(v_0 - v_deseada_0)+kappa_desired_0-kappa_0;
sum_result = eta1 + theta1*(v_0 - v_deseada_0)-kappa_desired_0 +kappa_0;

== matlab function ASG_algorithm/Subsystem1/MATLAB Function2 ==
  data: angles_vector input; R output; anglesdot_vector input; R_dot output; R_ddot output; anglesddot_vector input
function [R, R_dot, R_ddot]= fcn(angles_vector, anglesdot_vector, anglesddot_vector)
R = zeros(3,3);
R_dot = zeros(3,3);
R_ddot= zeros(3,3);

phi = angles_vector(1);
theta = angles_vector(2);
psi = angles_vector(3);


phi_dot = anglesdot_vector(1);
theta_dot = anglesdot_vector(2);
psi_dot = anglesdot_vector(3);

phi_ddot = anglesddot_vector(1);
theta_ddot = anglesddot_vector(2);
psi_ddot = anglesddot_vector(3);


 R = [ cos(theta)*cos(psi), cos(psi)*sin(phi)*sin(theta) - cos(phi)*sin(psi) , sin(phi)*sin(psi)+cos(phi)*cos(psi)*sin(theta);
       cos(theta)*sin(psi), cos(phi)*cos(psi) + sin(phi)*sin(theta)*sin(psi) , cos(phi)*sin(theta)*sin(psi)-cos(psi)*sin(phi);
       -sin(theta) , cos(theta)*sin(phi) , cos(phi)*cos(theta)];

 R_dot = -[0      -psi_dot theta_dot;
           psi_dot 0    -phi_dot;
           -theta_dot phi_dot 0 ] * R;

 matrix_aux =  [0      -psi_dot theta_dot;
           psi_dot 0    -phi_dot;
           -theta_dot phi_dot 0 ];

 R_ddot = (-[0      -psi_ddot theta_ddot;
           psi_ddot 0    -phi_ddot;
           -theta_ddot phi_ddot 0 ]   +  matrix_aux^2 )* R;

== matlab function ASG_algorithm/MATLAB Function6 ==
  data: delta1 input; s1 output; delta1_dot input; eta1 input; t input; theta1 input; a1x_average input; t_s1 output; a1y_average input; a1z_average input; Z1 output; norm_s1 output
function [s1, t_s1, Z1, norm_s1]= fcn(delta1, delta1_dot, eta1,t,theta1, a1x_average, a1y_average, a1z_average)
t_s1 = t; 
s1 = zeros(3,1);
Z1 = zeros(3,1);
s1 = delta1_dot+(delta1+eta1)/(t+theta1)-[a1x_average; a1y_average; a1z_average];
Z1 =[a1x_average; a1y_average; a1z_average];
norm_s1 = norm(s1);

== matlab function ASG_algorithm/MATLAB Function14 ==
  data: v_dot output; fv input; I_zero input; D_inv input; Q input; xi_subv input
function v_dot  = fcn(fv, I_zero, D_inv, Q, xi_subv)
v_dot = zeros(3,1);
v_dot=fv+I_zero*D_inv*Q+xi_subv;

== matlab function ASG_algorithm/eta2 ==
  data: theta2 input; eta2 output; THETA_0 input; THETA_deseada_0 input; THETA_DOT_desired_0 input; THETA_DOT_0 input; sum_result output
function [eta2, sum_result] = fcn(theta2,THETA_0, THETA_deseada_0, THETA_DOT_desired_0, THETA_DOT_0)
eta2 = -theta2*(THETA_DOT_0 - THETA_DOT_desired_0)+THETA_deseada_0-THETA_0;
sum_result = eta2+theta2*(THETA_DOT_0-THETA_DOT_desired_0)-THETA_deseada_0 +THETA_0;

== matlab function ASG_algorithm/MATLAB Function17 ==
  data: omega_dot output; fw input; zero_I input; D_inv input; Q input; xi_subw input
function omega_dot  = fcn(fw, zero_I, D_inv, Q, xi_subw)
omega_dot=zeros(3,1);
omega_dot=fw+zero_I*D_inv*Q+xi_subw;

== matlab function ASG_algorithm/MATLAB Function18 ==
  data: fw input; h_omega output; omega input; delta2 input; eta2 input; zeta2 input; theta2 input; t input; a2 input; D_inv input; Q input; zero_I input
function h_omega = fcn(fw,omega,delta2,eta2,zeta2,theta2,t,a2, D_inv, Q, zero_I)
h_omega = zeros(3,1);
%h_omega=w_dot+omega/(t+theta2)-a2/(t+theta2)-(delta2+eta2)/(t+theta2)^2+zeta2/(t+theta2)^2;
h_omega = fw+ omega/(t+theta2) -a2/(t+theta2) - (delta2+eta2)/(t+theta2)^2 + zeta2/(t+theta2)^2;

== matlab function ASG_algorithm/MATLAB Function9 ==
  data: D output; D_inv output; C output; g_q output; I_zero output; zero_I output; Ka input; drag_matrix output; l_arm output; M output; g output
function [D, D_inv, C, g_q, I_zero, zero_I,drag_matrix, l_arm, M,g] = fcn(Ka)
D_inv = zeros(6,6);
D = zeros(6,6);
drag_matrix = zeros(6,6);
g_q =zeros(6,1);
I_zero = zeros(3,6);
zero_I  = zeros(3,6);
l_arm = zeros(1,1);

g = 9.81;
 
m1_box = 0.532 ;
m2_arm =0.006 ;
m3_landingv =0.009 ;
m4_landingh =0.003;
M = m1_box + 4*m2_arm + 2*m3_landingv + 2*m4_landingh ;

delta_angle = 45;

h = 0.028 ;
l1 = 0.144;
l2 = 0.1485;
l3 = 0.3040;
l4 = 0.25 ;
d2 = (l1/sqrt(2) + l2/2)/sqrt(2);
d4_2 = (l1/2)^2+(l4/2*sin(delta_angle))^2; %d4^2
l_arm = l1/sqrt(2) + l2;

D=[M 0 0 m3_landingv*l3*sin(delta_angle) 2*m4_landingh*l3*sin(delta_angle) m3_landingv*(l3/2*cos(delta_angle)+(l1/2))-4*m2_arm*d2;
   0 M 0 -m3_landingv*l3*sin(delta_angle) 0 4*m2_arm*d2;
   0 0 M 4*m2_arm*d2+m3_landingv*(l3*cos(delta_angle)+l1) -4*m2_arm*d2 0;
   m3_landingv*l3*sin(delta_angle) -m3_landingv*l3*sin(delta_angle) 4*m2_arm*d2+m3_landingv*(l3*cos(delta_angle)+l1) (m1_box*l1^2+m2_arm*l1^2)/6+2*m3_landingv*(l3^2/3)+2*m4_landingh*(l4^2/12+d4_2) 0 0;
   2*m4_landingh*l3*sin(delta_angle) 0 -4*m2_arm*d2 0 (m1_box*l1^2+m2_arm*l1^2)/6+2*m3_landingv*(l3^2/3)*cos(delta_angle).^2+2*m4_landingh*(l4^2/12+d4_2) -2*m3_landingv*sin(delta_angle)*cos(delta_angle)*(l3^2/3);
   m3_landingv*(l3/2 * cos(delta_angle)+ l1/2)-4*m2_arm*d2 4*m2_arm*d2 0 0 -2*m3_landingv*sin(delta_angle)*cos(delta_angle)*(l3^2/3) m1_box*l1^2/6+4*m2_arm*((l2^2/12)+(h/sqrt(2)+h/2)^2)+2*m3_landingv*(l3^2/3*cos(delta_angle).^2+(l3^2/2*cos(delta_angle)+l1^2/2))+2*m4_landingh*d4_2
   ];

 D_inv = pinv(D);

    C=[-2*m4_landingh*l3*sin(delta_angle) 0 0 0 0 0;
        0 -2*m4_landingh*l4 0 0 0 0;
        0 0 2*m4_landingh*l4 0 -4*m2_arm*d2-2*m4_landingh*l4 0;
        0 0 0 0 0 0;
        0 0 0 0 0 0;
        0 0 0 0 0 0];

    g_q= [0; %vector gravitacional 
        0;
        M*g;
        0;
        0;
        0];

I_zero = [eye(3) zeros(3,3)] ;
zero_I = [zeros(3,3),eye(3)];
drag_matrix= [diag([Ka Ka Ka]) zeros(3,3); zeros(3,6)];

== matlab function ASG_algorithm/MATLAB Function19 ==
  data: delta2 input; s2 output; delta2_dot input; eta2 input; t input; theta2 input; a2x_average input; a2y_average input; a2z_average input; Z2 output; norm_s2 output
function [s2, Z2, norm_s2]= fcn(delta2, delta2_dot, eta2,t,theta2, a2x_average, a2y_average, a2z_average)
s2 = zeros(3,1);
Z2 = zeros(3,1);
s2 = delta2_dot+(delta2+eta2)/(t+theta2)-[a2x_average; a2y_average; a2z_average];
Z2 =[a2x_average; a2y_average; a2z_average];
norm_s2 = norm(s2);

== matlab function ASG_algorithm/MATLAB Function8 ==
  data: theta_actual input; delta2 output; delta2_dot output; a2 output; theta_desired input; F_d2 output; epsilon input; omega_actual input; omega_desired input; a2_x output; a2_y output; a2_z output
function [delta2, delta2_dot,a2, F_d2, a2_x, a2_y, a2_z] = fcn(theta_actual, theta_desired,  epsilon, omega_actual, omega_desired)
delta2=theta_actual-theta_desired;
delta2_dot=omega_actual-omega_desired;
F_d2=norm(delta2);
if F_d2 < epsilon
    a2 = zeros(3,1);
else
a2 = -delta2;  %quite el signo /F_d2
end
a2_x = a2(1);
a2_y = a2(2);
a2_z = a2(3);

== matlab function ASG_algorithm/MATLAB Function12 ==
  data: u1 output; D input; sign_s1 input; sign_s2 input; k1 input; h_v input; h_omega input; k2 input; s1 input; s2 input; value_s1 output; value_s2 output
function [u1, value_s1, value_s2 ]= fcn( D, sign_s1, sign_s2, k1, h_v,h_omega, k2, s1, s2)
u1 = zeros(6,1);

%u1 =D*(-[h_v;h_omega]-[k1*sign_s1;k2*sign_s2]);
value_s1 =zeros(3,1);
value_s2 =zeros(3,1);

for i=1:3 
    value_s1(i)= s1(i)/(abs(s1(i))+0.05) ; %(abs(s1(i))+0.05);
    value_s2(i)= s2(i)/(abs(s2(i))+0.05) ;   %(abs(s2(i))+0.05)
end
%s1(1)/(abs(s1(1))+0.0001) 

u1 =D*(-[h_v;h_omega]-[k1*value_s1;k2*value_s2 ]);

== matlab function ASG_algorithm/Enabled Subsystem/MATLAB Function ==
  data: v_actual_0 output; v_actual input; kappa_bar_0 output; kappa input; v_desired input; v_deseada_0 output; kappa_try input; kappa0 output; theta_actual input; omega_actual input; tetha0 output; theta_dot0 output; theta_desired input; thetadot_desired input; theta_desired0 output; thetadot_desired0 output
function [v_actual_0, kappa_bar_0, v_deseada_0, kappa0, tetha0, theta_dot0, theta_desired0, thetadot_desired0]= fcn(v_actual, kappa, v_desired, kappa_try, theta_actual, omega_actual, theta_desired, thetadot_desired)
kappa_bar_0 = kappa;
v_actual_0 = v_actual;
v_deseada_0 = v_desired;
kappa0 = kappa_try;  % x =0 , y=0, z = z+1 [kappa_try(1);kappa_try(2);kappa_try(3)+1];
tetha0=theta_actual;
theta_dot0=omega_actual;
theta_desired0 = theta_desired;
thetadot_desired0= thetadot_desired;

== matlab function ASG_algorithm/MATLAB Function28 ==
  data: omega_dot output; fw input; zero_I input; D_inv input; Q input; xi_subw input
function omega_dot  = fcn(fw, zero_I, D_inv, Q, xi_subw)
omega_dot=zeros(3,1);
omega_dot=fw+zero_I*D_inv*Q+xi_subw;

== matlab function ASG_algorithm/Subsystem1/MATLAB Function13 ==
  data: R input; R_six output; R_dot input; R_ddot input; R_dotsix output; R_ddotsix output
function [R_six, R_dotsix, R_ddotsix] = fcn(R, R_dot , R_ddot)
R_six = zeros(6,6);
R_dotsix = zeros(6,6);
R_ddotsix = zeros(6,6);

R_six = [R, zeros(3,3); 
        zeros(3,3), eye(3)];

R_dotsix = [R_dot, zeros(3,3); 
        zeros(3,3), eye(3)];

R_ddotsix = [R_ddot, zeros(3,3); 
        zeros(3,3), eye(3)];

== matlab function ASG_algorithm/Subsystem1/MATLAB Function1 ==
  data: Q_actual input; delta3 output; delta3_dot output; a3 output; Q_desired input; F_d3 output; epsilon input; Qdot_actual input; Qdot_desired input; a3_x output; a3_y output; a3_z output; a3_phi output; a3_theta output; a3_psi output; alpha input; k31 input
function [delta3, delta3_dot,a3, F_d3, a3_x, a3_y, a3_z, a3_phi, a3_theta, a3_psi] = fcn(Q_actual, Q_desired,  epsilon, Qdot_actual, Qdot_desired, alpha, k31)
delta3 = zeros(6,1);
delta3_dot= zeros(6,1);

a3_x = zeros(1,1);
a3_y = zeros(1,1);
a3_z = zeros(1,1);
a3_phi = zeros(1,1);
a3_theta = zeros(1,1);
a3_psi = zeros(1,1);
F_d3 = zeros(1,1);
a3 = zeros(6,1);

delta3= Q_actual-Q_desired;
delta3_dot=Qdot_actual-Qdot_desired;

F_d3=1/2*norm(delta3)^2;

if F_d3 < epsilon
    a3 = zeros(6,1);
else
a3 = alpha*k31*delta3;  %quite el signo /F_d3
end

a3_x = a3(1);
a3_y = a3(2);
a3_z = a3(3);
a3_phi   = a3(4);
a3_theta = a3(5);
a3_psi   = a3(6);

== matlab function ASG_algorithm/MATLAB Function20 ==
  data: t input; kappa output
function kappa = fcn(t)
    % Parámetros de la elipse
    w = 1;    % Velocidad angular
    a = 25;  %5 25  % Semieje mayor (eje x)
    b = 15;    %3 15 Semieje menor (eje y)
    x0 = 0;   % Centro en x
    y0 = 0;   % Centro en y
    z0 = 20;   % Altura inicial (eje z)

    % Ángulos de inclinación (en radianes)
    theta_x = 0;  % 30° de inclinación alrededor del eje X
    theta_y = pi/6; % 15° de inclinación alrededor del eje Y

    % Ecuaciones paramétricas originales (elipse en plano XY)
    x_t = a * cos(w * t);
    y_t = b * sin(w * t);
    z_t = 0;  % Elipse inicialmente en z=0

    % Matrices de rotación
    Rx = [1      0           0;
          0 cos(theta_x) -sin(theta_x);
          0 sin(theta_x)  cos(theta_x)];

    Ry = [cos(theta_y)  0 sin(theta_y);
               0       1      0;
          -sin(theta_y) 0 cos(theta_y)];

    % Rotar la elipse (primero X, luego Y)
    rotated_point = Ry * Rx * [x_t; y_t; z_t];

    % Trasladar al centro deseado (x0, y0, z0)
    kappa = rotated_point + [x0; y0; z0];
end

== matlab function ASG_algorithm/MATLAB Function21 ==
  settings: updateMethod=DISCRETE
  data: des_vel input; desired_theta output
function desired_theta = fcn(des_vel)
desired_theta = zeros(3,1);

    % Extraer velocidades
    vx = des_vel(1);
    vy = des_vel(2);
    vz = des_vel(3);

    %---------------------------
    % RAW YAW (salta en ±pi)
    psi_raw = atan2(vy, vx);

 persistent prev_vec psi_accum_internal
    if isempty(prev_vec)
        prev_vec = [1; 0];          % orientación inicial hacia X+
        psi_accum_internal = 0;
    end

    % Vector de dirección actual (normalizado)
    curr_vec = [vx; vy];
    curr_norm = norm(curr_vec);
    if curr_norm < 1e-6
        curr_vec = prev_vec;  % si está casi detenido, no actualizamos
    else
        curr_vec = curr_vec / curr_norm;
    end

    % Producto cruzado (z) y escalar (dot)
    cross_z = prev_vec(1)*curr_vec(2) - prev_vec(2)*curr_vec(1);
    dot_val = prev_vec(1)*curr_vec(1) + prev_vec(2)*curr_vec(2);

    delta_psi = atan2(cross_z, dot_val);
    psi_accum_internal = psi_accum_internal + delta_psi;

    % Actualiza vector anterior
    prev_vec = curr_vec;
    psi_accum = psi_accum_internal;

    %---------------------------
    % PITCH
    horizontal_speed = sqrt(vx^2 + vy^2);
    theta = atan(vz / (horizontal_speed + 1e-6));

    % ROLL (fijo)
    phi = 0;

    %---------------------------
    % Salida principal
    %desired_theta = [phi; theta; psi_accum];
    desired_theta = [0; 0; 0];

== matlab function ASG_algorithm/Subsystem1/AverageBlock6/MATLAB Function ==
  data: t input; t_plus_theta output; theta input
function t_plus_theta = fcn(t, theta)
t_plus_theta = 1/(t+theta);
